simulink model "pid_regulator"  (R2019b)
settings: Solver=VariableStepAuto  StartTime=0.0  StopTime=2  MaxStep=0.005  MinStep=0.001  RelTol=0.001  AbsTol=0.005
undefined symbols (not defined in the file): J, km, L, R
settings Model: Creator=Gudini  LastModifiedBy=Gudini
settings SolverCC: InitialStep=0.002  MaxConsecutiveMinStep=5

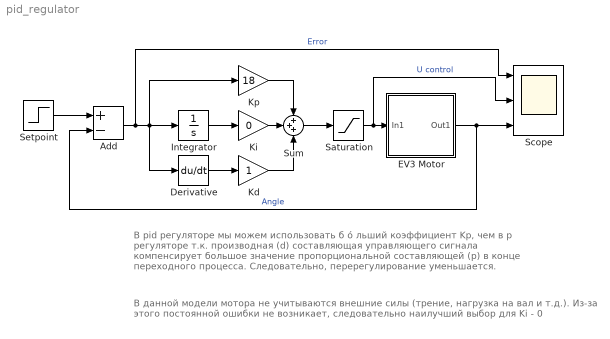
== system pid_regulator ==
  note: В данной модели мотора не учитываются внешние силы (трение, нагрузка на вал и т.д.).
      |  Из-за этого постоянной ошибки не возникает, следовательно наилучший выбор для Ki - 0
  note: В pid регуляторе мы можем использовать б ó льший коэффициент Kp,
      | чем в p регуляторе т.к. производная (d) составляющая управляющего сигнала
      | компенсирует большое значение пропорциональной составляющей (p) в конце
      | переходного процесса. Следовательно, перерегулирование уменьшается.
  Add : Sum  Inputs=+-
  Derivative : Derivative
  EV3 Motor : Subsystem
  Integrator : Integrator  AbsoluteTolerance=0.05
  Kd : Gain
  Ki : Gain  Gain=0
  Kp : Gain  Gain=18
  Saturation : Saturate  UpperLimit=7.6  LowerLimit=-7.6  ZeroCross=off
  Scope : Scope  NumInputPorts=3
  "Setpoint " : Step  Time=0.2  After=3.14  SampleTime=0
  Sum : Sum  Inputs=+++
  wires:
  Saturation/1 -> Scope/2, EV3 Motor/1(In1)  "U control"
  "Setpoint "/1 -> Add/1
  EV3 Motor/1(Out1) -> Add/2, Scope/3  "Angle"
  Ki/1 -> Sum/2
  Kd/1 -> Sum/3
  Kp/1 -> Sum/1
  Integrator/1 -> Ki/1
  Derivative/1 -> Kd/1
  Add/1 -> Scope/1, Derivative/1, Kp/1, Integrator/1  "Error"
  Sum/1 -> Saturation/1

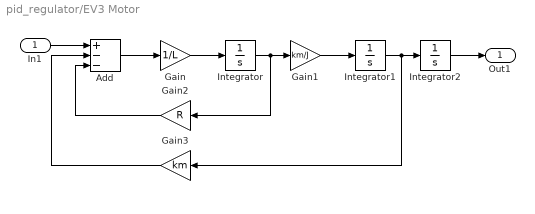
== system pid_regulator/EV3 Motor ==
  In1 : Inport
  Add : Sum  Inputs=+--
  Gain : Gain  Gain=1/L
  Gain1 : Gain  Gain=km/J
  Gain2 : Gain  Gain=R
  Gain3 : Gain  Gain=km
  Integrator : Integrator
  Integrator1 : Integrator
  Integrator2 : Integrator
  Out1 : Outport
  wires:
  Gain1/1 -> Integrator1/1
  Integrator1/1 -> Gain3/1, Integrator2/1
  In1/1 -> Add/1
  Integrator2/1 -> Out1/1
  Integrator/1 -> Gain2/1, Gain1/1
  Gain/1 -> Integrator/1
  Gain2/1 -> Add/3
  Add/1 -> Gain/1
  Gain3/1 -> Add/2
